simulink model "sfbuilder_multiport"  (Simulink 6.0)
settings: Solver=ode1  SolverMode=SingleTasking  StartTime=0.0  StopTime=10.0  RelTol=1e-3
settings Model: Creator=The MathWorks Inc.  LastModifiedBy=batserve  ExtModeAutoUpdateStatusClock=off
settings DataIOCC: SignalLoggingName=sigsOut
settings OptimizationCC: BooleanDataType=off
settings DebuggingCC: CheckExecutionContextPreStartOutputMsg=on  CheckExecutionContextRuntimeOutputMsg=on  SolverPrmCheckMsg=none
settings HardwareCC: TargetUnknown=on

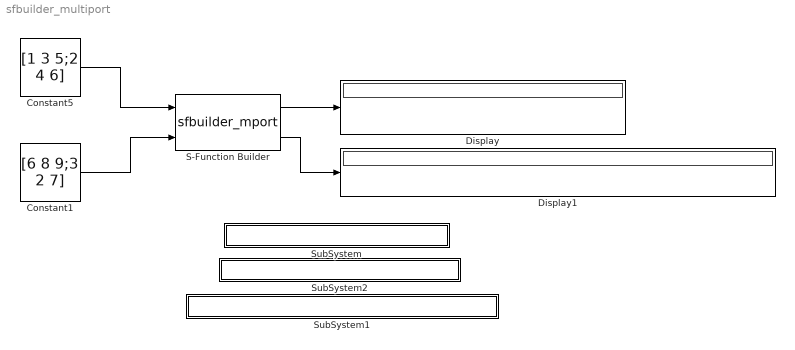
== system sfbuilder_multiport ==
  Constant1 : Constant  Value=[6 8 9;3 2 7]  VectorParams1D=off  OutDataTypeMode=int32
  Constant5 : Constant  Value=[1 3 5;2 4 6]  VectorParams1D=off  OutDataTypeMode=single
  Display : Display
  Display1 : Display
  S-Function Builder : S-Function  FunctionName=sfbuilder_mport  SFunctionModules=sfbuilder_mport_wrapper  WizardData=DataTag0  mask(S-Function Builder){}
      mask init:
      | val = [[.9  0.75 0.75 1 1 .9 .9 1]',[1 1 0.75 0.75 .9 .9 1 .9]'];
      | sys = get_param(gcb,'FunctionName');
      settings: CopyFcn=set_param(gcb,'LinkStatus','none')  OpenFcn=sfunctionwizard(gcbh)
      mask Display:
      | plot(val(:,1),val(:,2))
      | disp(sys)
      | port_label('input',1,'in1')
      | port_label('input',2,'in2')
      | port_label('output',1,'out1')
      | port_label('output',2,'out2')
  SubSystem : Subsystem  PropExecContextAcrossSSBoundary=on
      settings: AttributesFormatString=\n\n  OpenFcn=edit(fullfile(matlabroot,'simulink','src','sfbuilder_mport.c'))
      mask Display: disp('matlabroot\simulink\src\sfbuilder_mport.c');
  SubSystem1 : Subsystem  PropExecContextAcrossSSBoundary=on
      settings: AttributesFormatString=\n\n  OpenFcn=edit(fullfile(matlabroot,'toolbox','simulink','blocks','tlc_c','sfbuilder_mport.tlc'))
      mask Display: disp('matlabroot\toolbox\simulink\blocks\tlc_c\sfbuilder_mport.tlc');
  SubSystem2 : Subsystem  PropExecContextAcrossSSBoundary=on
      settings: AttributesFormatString=\n\n\n  OpenFcn=edit(fullfile(matlabroot,'simulink','src','sfbuilder_mport_wrapper.c'))
      mask Display: disp('matlabroot\simulink\src\sfbuilder_mport_wrapper.c');
  wires:
  Constant1/1 -> S-Function Builder/2
  Constant5/1 -> S-Function Builder/1
  S-Function Builder/1 -> Display/1
  S-Function Builder/2 -> Display1/1

== system sfbuilder_multiport/SubSystem ==

== system sfbuilder_multiport/SubSystem1 ==

== system sfbuilder_multiport/SubSystem2 ==
